simulink model "three_phase_uncontrolled_converter"  (R2023b)
settings: Solver=ode23t  StartTime=0.0  StopTime=0.2  RelTol=1e-3
libraries: spsDiodeLib x6, spsVoltageMeasurementLib x4, spsCurrentMeasurementLib x2, spsSeriesRLCBranchLib x1, spsThreePhaseSourceLib x1, sps_lib x1
settings Model: Creator=nandhitha  LastModifiedBy=essa7

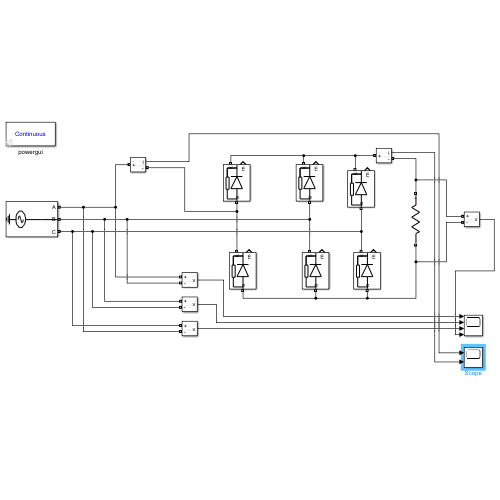
[thumbnail: Simulink's stored preview of the top-level diagram]
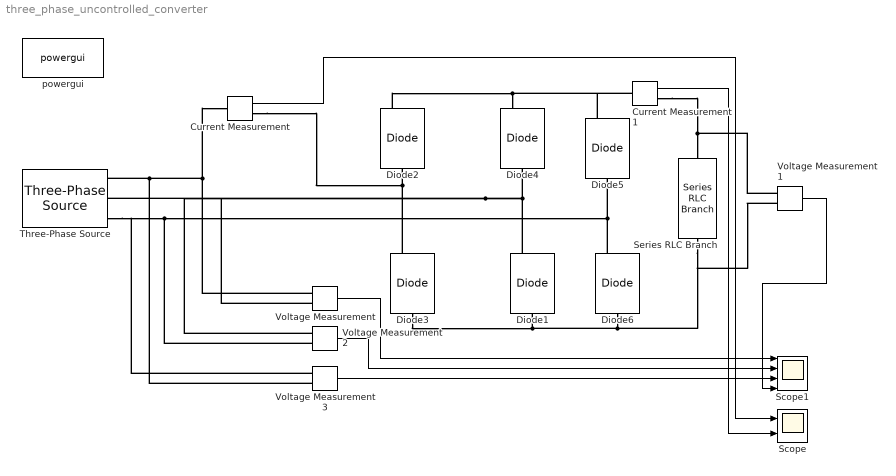
== system three_phase_uncontrolled_converter ==
  Current Measurement : spsCurrentMeasurementLib/Current Measurement  PhasorSimulation=off  OutputType=Complex  PSBequivalent=0
  Current Measurement1 : spsCurrentMeasurementLib/Current Measurement  PhasorSimulation=off  OutputType=Complex  PSBequivalent=0
  Diode{1..6} (6 alike) : spsDiodeLib/Diode  Ron=0.001  Lon=0  Vf=0.8  IC=0  UseSnubber=0  Rs=500  Cs=250e-9  Measurements=on
  Scope : Scope  NumInputPorts=2
  Scope1 : Scope  NumInputPorts=4
  Series RLC Branch : spsSeriesRLCBranchLib/Series RLC Branch  LConnTagsString=__new0  RConnTagsString=__new0  BranchType=R  Resistance=2  Inductance=1e-3  SetiL0=off  InitialCurrent=0  Capacitance=1e-6  Setx0=off  InitialVoltage=0  Measurements=None
  Three-Phase Source : spsThreePhaseSourceLib/Three-Phase Source  InternalConnection=Yg  VoltagePhases=off  Voltage=230  PhaseAngle=0  Voltage_phases=[25e3 25e3 25e3]/sqrt(3)  PhaseAngles_phases=[0 -120 +120]  Frequency=50  NonIdealSource=off  SpecifyImpedance=off  Resistance=0  Inductance=0  ShortCircuitLevel=100e6  BaseVoltage=230  XRratio=7  BusType=swing  Pref=10e3  Qref=0  Prefabc=[10e3, 10e3, 10e3]  Qrefabc=[0, 0, 0]  Qmin=-inf  Qmax=inf
  Voltage Measurement{,1..3} (4 alike) : spsVoltageMeasurementLib/Voltage Measurement  PhasorSimulation=off  OutputType=Complex  PSBequivalent=0
  powergui : sps_lib/powergui  Priority=1  SimulationMode=Continuous  SampleTime=50e-6  frequency=60  Iterations=50  frequencyindice=50  Pbase=100e6  ErrMax=1e-4  UnitsV=kV  UnitsW=MW  buscounter=0  FunctionMessages=off  echomessages=off  EnableUseOfTLC=off  CurrentSourceSwitches=off  DisableSnubberDevices=off  DisableRonSwitches=off  DisableVfSwitches=off  DisplayEquations=off  AutomaticDiscreteSolvers=off  SolverType=Tustin/Backward Euler (TBE)  Interpol=off  ExternalGateDelay=off  methode=off  Ts=100  x0status=blocks  SPID=on  SwTol=0  HookPort=off  NonlinearTolerance=1e-4  nMaxIteration=100  ContinueOnMaxIteration=off  RestoreLinks=warning  ResistiveCurrentMeasurement=off  Frange=[0:2:500]  Ylog=off  Xlog=on  ShowGrid=off  save=off  variable=ZData  structure=0  ZoomFFT=off  StartTime=0.0  cycles=1  DisplayStyle=1  fundamental=60  FreqAxis=off  MaxFrequency=1000  frequencyindicesteady=1  RmsSteady=1  display=off
  wires:
  Current Measurement/1 -> Scope/1
  Voltage Measurement/1 -> Scope1/1
  Voltage Measurement1/1 -> Scope1/4
  Current Measurement1/1 -> Scope/2
  Voltage Measurement2/1 -> Scope1/2
  Voltage Measurement3/1 -> Scope1/3
  connections:
  Diode3/LConn1 -- Diode6/LConn1 -- Series RLC Branch/RConn1 -- Voltage Measurement1/LConn2 -- Diode1/LConn1
  Diode1/RConn1 -- Voltage Measurement/LConn2 -- Voltage Measurement2/LConn1 -- Three-Phase Source/RConn2 -- Diode4/LConn1
  Diode2/RConn1 -- Diode5/RConn1 -- Current Measurement1/LConn1 -- Diode4/RConn1
  Current Measurement1/RConn1 -- Voltage Measurement1/LConn1 -- Series RLC Branch/LConn1
  Diode3/RConn1 -- Current Measurement/RConn1 -- Diode2/LConn1
  Voltage Measurement/LConn1 -- Current Measurement/LConn1 -- Voltage Measurement3/LConn2 -- Three-Phase Source/RConn1
  Diode6/RConn1 -- Voltage Measurement2/LConn2 -- Three-Phase Source/RConn3 -- Voltage Measurement3/LConn1 -- Diode5/LConn1
